simulink model "mfcncalloutput"  (Simulink 6.1)
settings: Solver=ode45  StartTime=0.0  StopTime=10.0  RelTol=1e-3
settings Model: Creator=mshakeri  LastModifiedBy=mshakeri  ExtModeAutoUpdateStatusClock=off
settings OptimizationCC: InlineParams=on  InlineInvariantSignals=off
settings DebuggingCC: SolverPrmCheckMsg=warning

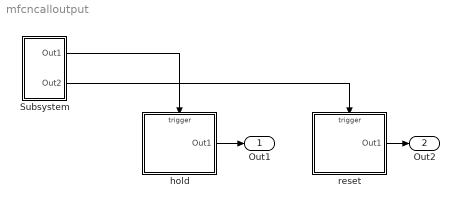
== system mfcncalloutput ==
  Subsystem : Subsystem  TreatAsAtomicUnit=on
  hold : Subsystem  TreatAsAtomicUnit=on
  reset : Subsystem  TreatAsAtomicUnit=on
  Out1 : Outport
  Out2 : Outport  Port=2
  wires:
  Subsystem/1(Out1) -> hold/Trigger
  Subsystem/2(Out2) -> reset/Trigger
  hold/1(Out1) -> Out1/1
  reset/1(Out1) -> Out2/1

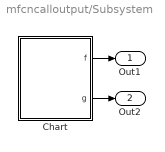
== system mfcncalloutput/Subsystem ==
  Chart : Stateflow chart
  Out1 : Outport
  Out2 : Outport  Port=2
  wires:
  Chart/1(f) -> Out1/1
  Chart/2(g) -> Out2/1

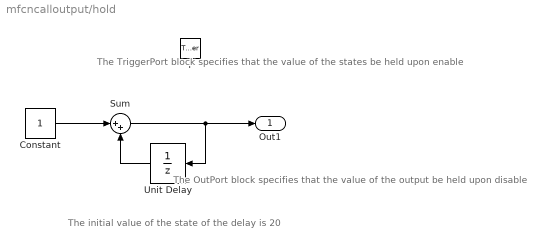
== system mfcncalloutput/hold ==
  note: The TriggerPort block
      | specifies that the value
      | of the states be held
      | upon enable
  note: The OutPort block
      | specifies that the value
      | of the output be held
      | upon disable
  note: The initial value of the state of the delay is 20
  f : TriggerPort  TriggerType=function-call
  Constant : Constant
  Sum : Sum  Inputs=|++  SaturateOnIntegerOverflow=on  InputSameDT=on
  Unit Delay : UnitDelay  Orientation=left  X0=20  SampleTime=-1
  Out1 : Outport
  wires:
  Constant/1 -> Sum/1
  Unit Delay/1 -> Sum/2
  Sum/1 -> Out1/1, Unit Delay/1

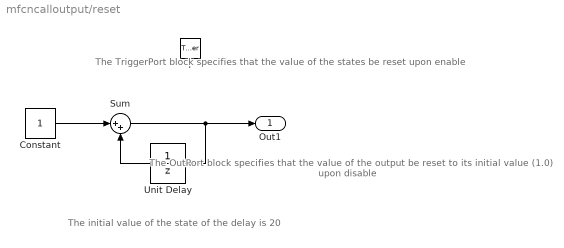
== system mfcncalloutput/reset ==
  note: The initial value of the state of the delay is 20
  note: The OutPort block
      | specifies that the value
      | of the output be reset
      | to its initial value (1.0)
      | upon disable
  note: The TriggerPort block
      | specifies that the value
      | of the states be reset
      | upon enable
  f : TriggerPort  TriggerType=function-call  StatesWhenEnabling=reset
  Constant : Constant
  Sum : Sum  Inputs=|++  SaturateOnIntegerOverflow=on  InputSameDT=on
  Unit Delay : UnitDelay  Orientation=left  X0=20  SampleTime=-1
  Out1 : Outport  OutputWhenDisabled=reset  InitialOutput=1
  wires:
  Sum/1 -> Unit Delay/1, Out1/1
  Unit Delay/1 -> Sum/2
  Constant/1 -> Sum/1

== stateflow chart Subsystem/Chart ==
  settings: updateMethod=DISCRETE  sampleTime=0.1
  state one/
    entry: f;
  state two/
    entry: g;
  one -> two
  two -> one
  (default) -> one
  events: f output FUNCTION_CALL_EVENT; g output FUNCTION_CALL_EVENT
